simulink model "lect2_pg18"  (R2024b)
settings: Solver=VariableStepAuto  StartTime=0.0  StopTime=10.0  RelTol=1e-3
settings Model: Creator=ramse  LastModifiedBy=ramse

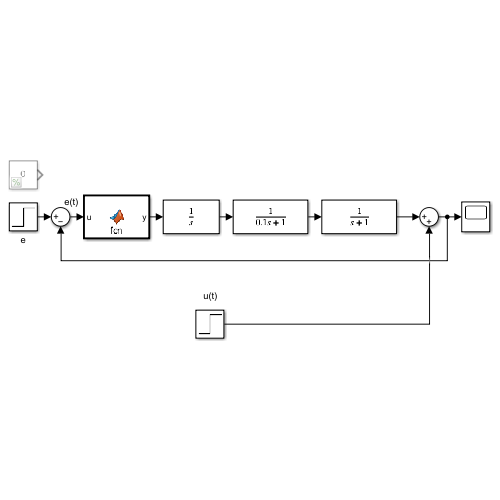
[thumbnail: Simulink's stored preview of the top-level diagram]
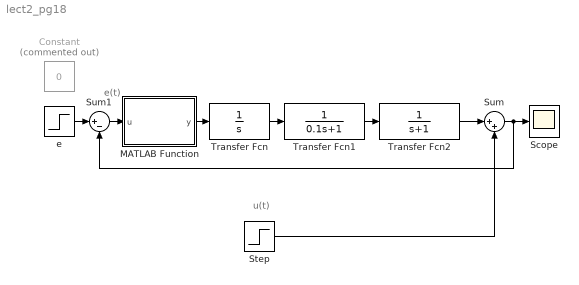
== system lect2_pg18 ==
  note: e(t)
  note: u(t)
  Constant : Constant  Commented=on  Value=0
  MATLAB Function : MATLAB Function  TreatAsAtomicUnit=on
  Scope : Scope
  Step : Step  SampleTime=0
  Sum : Sum  Inputs=|++
  Sum1 : Sum  Inputs=|+-
  Transfer Fcn : TransferFcn  Denominator=[1 0]
  Transfer Fcn1 : TransferFcn  Denominator=[0.1, 1]
  Transfer Fcn2 : TransferFcn  Denominator=[1, 1]
  e : Step  SampleTime=0
  wires:
  Transfer Fcn/1 -> Transfer Fcn1/1
  Transfer Fcn1/1 -> Transfer Fcn2/1
  MATLAB Function/1(y) -> Transfer Fcn/1
  Transfer Fcn2/1 -> Sum/1
  Sum/1 -> Sum1/2, Scope/1
  e/1 -> Sum1/1
  Sum1/1 -> MATLAB Function/1(u)
  Step/1 -> Sum/2

== matlab function lect2_pg18/MATLAB Function ==
  data: u input; y output
function y = fcn(u)
k=1;
a=1;

if u>a
    y=k*a;
elseif (-a<u)&&(u<a)
    y=k*u;
else
    y=k*a;
end
